simulink model "Lab5_Q3"  (R2021a)
settings: Solver=FixedStepDiscrete  StartTime=0.0  StopTime=10.0  FixedStep=1e-5  RelTol=1e-3
settings Model: Creator=student  LastModifiedBy=student

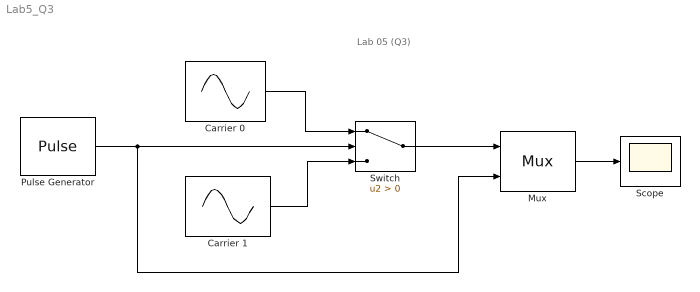
== system Lab5_Q3 ==
  note: Lab 05 (Q3)
  Carrier 0 : Sin  Frequency=3141.5926  SampleTime=0.01
  Carrier 1 : Sin  Frequency=9424.7779  SampleTime=0.01
  Mux : Mux  Inputs=2
  Pulse Generator : DiscretePulseGenerator  PulseType=Time based  Period=0.001  PulseWidth=50
  Scope : Scope
  Switch : Switch  Criteria=u2 > Threshold
  wires:
  Carrier 0/1 -> Switch/1
  Pulse Generator/1 -> Mux/2, Switch/2
  Switch/1 -> Mux/1
  Mux/1 -> Scope/1
  Carrier 1/1 -> Switch/3
